simulink model "battery_PV_microgrid"  (R2014a)
settings: Solver=ode23tb  StartTime=0.0  StopTime=86000  MaxStep=0.2  RelTol=1e-5
InitFcn:
  | % Load Stateflow/Controller Parameters
  | controlParams();
  | 
  | % Load Initial Conditions for Model
  | initialConditions();
  | 
  | % Load Battery/PV Parameters
  | parameters();
StopFcn:
  | % Plot results
  | %plotSimResults();
values from neighbouring files (symbols this model uses):
  ambientTemp = 20    [initialConditions.m]    (also in initializeBattery.m)
  currentSat = 0.5    [controlParams.m]    (also in initializeBattery.m)
  desiredBusVoltage = 30    [controlParams.m]    (also in initializeBattery.m = 24.45)
  finalVoltage = 30    [controlParams.m]    (also in initializeBattery.m = 26)
  maxChargeRate = 5    [controlParams.m]    (also in initializeBattery.m)
  maxDischargeRate = -5    [controlParams.m]    (also in initializeBattery.m)
  Ncell = 100    [parameters.m]
  T_init = ambientTemp + 273.15    (= 293.15)    [initialConditions.m]    (also in initializeBattery.m)
  tau = 1e-4    (= 0.0001)    [parameters.m]
undefined symbols (not defined in the file or in its folder): hysteresisSOC, Ion, Lithium, maxSOC, minSOC, optTime, powerHysteresis
undefined symbols (not defined in the file): C1_LUT, C2_LUT, Capacity_LUT, cell_Cp_heat, cell_mass, Em_LUT, PVCellIsc, PVCellRs, PVCellVoc, Qe_init, R0_LUT, R1_LUT, R2_LUT, SOC_LUT, Temperature_LUT
libraries: powerlib x49, fl_lib x18, nesl_utility x6, LiBatteryElements_lib x6, simulink x3, simulink_extras x3, electricdrivelib x1
(part 1 of 2)
settings Model: Creator=jlesage  LastModifiedBy=jlesage
settings DataIOCC: LimitDataPoints=off
settings DebuggingCC: MergeDetectMultiDrivingBlocksExec=error
settings SimscapeCC: ExplicitSolverDiagnosticOptions=none

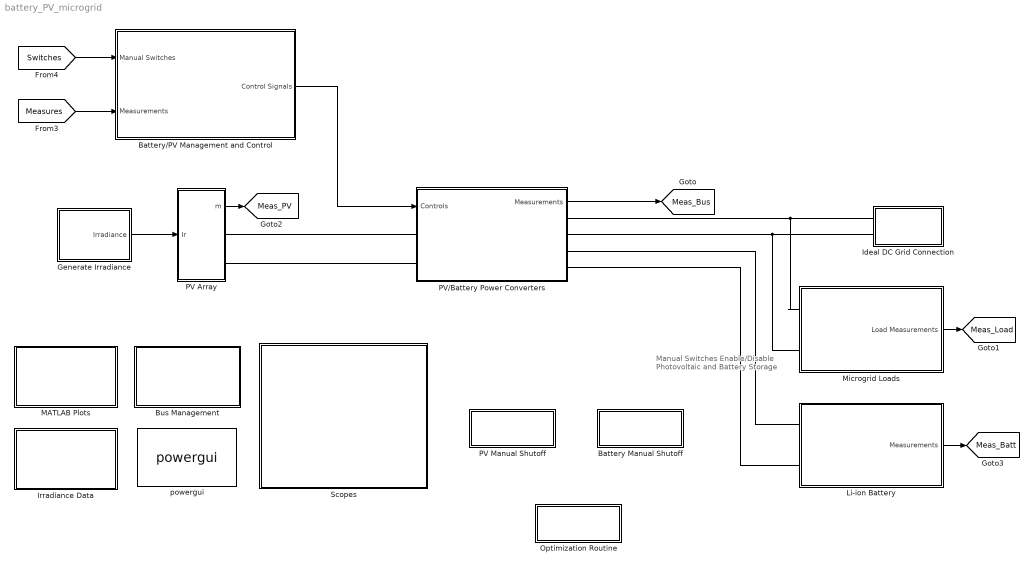
== system battery_PV_microgrid ==
  note: Manual Switches
      | Enable/Disable Photovoltaic
      | and Battery Storage
  Battery Manual Shutoff : Subsystem
      settings: OpenFcn=|
      | blkName = gcb;
      | switchBlkName = [gcb '/ControlValue'];
      | 
      | switchValue = get_param(switchBlkName,'Value');
      | switchValue = str2num(switchValue);
      | 
      | if switchValue > 0,
      | 
      | set_param(switchBlkName,'Value','-1');
      | set_param(blkName,'BackgroundColor','red');
      | set_param(blkName,'MaskDisplay','disp(''Battery On/Off\nOFF'')');
      | 
      | else
      | 
      | set_param(switchBlkName,'Value','1');
      | set_param(blkName,'BackgroundColor','green');
      | set_param(blkName,'MaskDisplay','disp(''Battery On/Off\nON'')');
      | 
      | 
      | end
      mask Display: disp('Battery On/Off\nON')
  Battery/PV Management and Control : Subsystem
  Bus Management : Subsystem
      mask Display: disp('Bus\nManagement');
  Generate Irradiance : Subsystem
  Ideal DC Grid Connection : Subsystem
  Irradiance Data : Subsystem
      settings: OpenFcn=|
      | blkName = gcb;
      | switchBlkName = [gcb '/ControlValue'];
      | 
      | switchValue = get_param(switchBlkName,'Value');
      | switchValue = str2num(switchValue);
      | 
      | if switchValue > 0,
      | 
      | set_param(switchBlkName,'Value','-1');
      | set_param(blkName,'MaskDisplay','disp(''Irradiance Data:\n Cloudy Day'')');
      | 
      | else
      | 
      | set_param(switchBlkName,'Value','1');
      | set_param(blkName,'MaskDisplay','disp(''Irradiance Data:\n Clear Day'')');
      | 
      | 
      | end
      mask Display: disp('Irradiance Data:\n Cloudy Day')
  Li-ion Battery : Subsystem  Variant=on  OverrideUsingVariant=Variant
  MATLAB Plots : Subsystem
      settings: OpenFcn=|
      | try
      | plotSimResults();
      | catch
      | disp('Run simulation before plotting results...');
      | end
      mask Display: disp('Plot Simulation\nResults');
  Microgrid Loads : Subsystem  Variant=on  OverrideUsingVariant=Variant
  Optimization Routine : Subsystem
      settings: OpenFcn=|
      | blkName = gcb;
      | switchBlkName = [gcb '/ControlValue'];
      | 
      | switchValue = get_param(switchBlkName,'Value');
      | switchValue = str2num(switchValue);
      | 
      | if switchValue > 0,
      | 
      | set_param(switchBlkName,'Value','-1');
      | set_param(blkName,'BackgroundColor','red');
      | set_param(blkName,'MaskDisplay','disp(''Optimization:\nOFF'')');
      | 
      | else
      | 
      | set_param(switchBlkName,'Value','1');
      | set_param(blkName,'BackgroundColor','green');
      | set_param(blkName,'MaskDisplay','disp(''Optimization:\nON'')');
      | 
      | 
      | end
      mask Display: disp('Optimization:\nOFF')
  PV Array : Subsystem
      mask Display: image(imread('panel.jpg'))
  PV Manual Shutoff : Subsystem
      settings: OpenFcn=|
      | blkName = gcb;
      | switchBlkName = [gcb '/ControlValue'];
      | 
      | switchValue = get_param(switchBlkName,'Value');
      | switchValue = str2num(switchValue);
      | 
      | if switchValue > 0,
      | 
      | set_param(switchBlkName,'Value','-1');
      | set_param(blkName,'BackgroundColor','red');
      | set_param(blkName,'MaskDisplay','disp(''PV On/Off\nOFF'')');
      | 
      | else
      | 
      | set_param(switchBlkName,'Value','1');
      | set_param(blkName,'BackgroundColor','green');
      | set_param(blkName,'MaskDisplay','disp(''PV On/Off\nON'')');
      | 
      | 
      | end
      mask Display: disp('PV On/Off\nON')
  PV/Battery Power Converters : Subsystem
  Scopes : Subsystem
      mask Display: disp('System\nMeasurements');
  powergui : powerlib/powergui  Priority=1  SimulationMode=Continuous  SolverType=Tustin  SampleTime=50e-6  frequency=60  SPID=on  DisableSnubberDevices=off  DisableRonSwitches=off  DisableVfSwitches=off  SwTol=0  Interpol=off  DisplayEquations=off  Ts=0  methode=off  frequencyindice=0  Pbase=100e6  ErrMax=1e-4  Iterations=50  UnitsV=kV  UnitsW=MW  FunctionMessages=off  echomessages=off  HookPort=off  EnableUseOfTLC=off  x0status=blocks  RestoreLinks=warning  ResistiveCurrentMeasurement=off  Frange=[0:2:500]  Ylog=off  Xlog=on  ShowGrid=off  save=off  variable=ZData  structure=0  ZoomFFT=off  StartTime=0.0  cycles=1  DisplayStyle=1  fundamental=60  FreqAxis=off  MaxFrequency=1000  frequencyindicesteady=1  RmsSteady=1  display=off
  tag scope: Meas_Batt=global, Meas_Bus=global, Meas_Load=global, Meas_PV=global
  wires:
  Microgrid Loads/1(Load Measurements) -> [Meas_Load]
  PV Array/1(m) -> [Meas_PV]
  Generate Irradiance/1(Irradiance) -> PV Array/1(Ir)
  Li-ion Battery/1(Measurements) -> [Meas_Batt]
  [Measures] -> Battery/PV Management and Control/2(Measurements)
  Battery/PV Management and Control/1(Control Signals) -> PV/Battery Power Converters/1(Controls)
  PV/Battery Power Converters/1(Measurements) -> [Meas_Bus]
  [Switches] -> Battery/PV Management and Control/1(Manual Switches)
  connections:
  Microgrid Loads/LConn2 -- PV/Battery Power Converters/RConn2 -- Ideal DC Grid Connection/LConn2
  Microgrid Loads/LConn1 -- PV/Battery Power Converters/RConn1 -- Ideal DC Grid Connection/LConn1
  PV Array/RConn1 -- PV/Battery Power Converters/LConn1
  PV Array/RConn2 -- PV/Battery Power Converters/LConn2
  PV/Battery Power Converters/RConn3 -- Li-ion Battery/LConn1
  Li-ion Battery/LConn2 -- PV/Battery Power Converters/RConn4

== system battery_PV_microgrid/Battery Manual Shutoff ==
  ControlValue : Constant
  Off : Constant  Value=0
  On : Constant
  Switch : Switch
  tag scope: BatterySwitch=global
  wires:
  Off/1 -> Switch/3
  ControlValue/1 -> Switch/2
  On/1 -> Switch/1
  Switch/1 -> [BatterySwitch]

== system battery_PV_microgrid/Battery//PV Management and Control ==
  Manual Switches : Inport
  Measurements : Inport  Port=2
  Battery Charge/Discharge Controllers : Subsystem
  Battery Mode Selection : Stateflow chart  TreatAsAtomicUnit=on
  Bus Creator : BusCreator  OutDataTypeStr=Bus: Controls
  Bus Selector : BusSelector  OutputSignals=pv
  Bus Selector1 : BusSelector  Commented=on  OutputSignals=opt
  MPPT Algorithm : Subsystem
  Optimization Routine : Subsystem  Commented=on  TreatAsAtomicUnit=on
  Signal Conversion : SignalConversion
  Control Signals : Outport
  tag scope: gridOnOff=global
  wires:
  Manual Switches/1 -> Bus Selector1/1, Bus Selector/1, Battery Mode Selection/1(switches)
  Battery Charge/Discharge Controllers/1(Duty) -> Bus Creator/3  "dutyBatt"
  Battery Mode Selection/1(controlOnOff) -> Battery Charge/Discharge Controllers/Enable, Bus Creator/2  "enableBatt"
  Bus Creator/1 -> Control Signals/1
  Battery Mode Selection/3(controlSelect) -> Battery Charge/Discharge Controllers/2(Controller Mode)
  Battery Mode Selection/2(batteryMode) -> Battery Charge/Discharge Controllers/1(Bus Switch)
  MPPT Algorithm/1(PV Duty) -> Bus Creator/4  "dutyPV"
  Bus Selector/1 -> Signal Conversion/1  "<pv>"
  Signal Conversion/1 -> Bus Creator/1  "enablePV"
  Battery Mode Selection/4(gridOnOff) -> [gridOnOff]
  Measurements/1 -> Optimization Routine/1(In1), MPPT Algorithm/1(Measurements), Battery Charge/Discharge Controllers/3(Measurements), Battery Mode Selection/2(measures)
  Bus Selector1/1 -> Optimization Routine/Enable  "<opt>"

== system battery_PV_microgrid/Bus Management ==
  note: Measurement Bus
  note: Manual Switch Bus
  note: ff
  note: ff
  note: Construct Measurement and Switch Buses
  Bus Creator : BusCreator  Inputs=5  OutDataTypeStr=Bus: Measurements
  Bus Creator1 : BusCreator  Inputs=3  OutDataTypeStr=Bus: Switches
  tag scope: Measures=global, Switches=global
  wires:
  [Meas_Load] -> Bus Creator/3  "load"
  [Meas_Bus] -> Bus Creator/2  "bus"
  Bus Creator/1 -> [Measures]
  [Meas_Batt] -> Bus Creator/5  "batt"
  [Meas_PV] -> Bus Creator/4  "pv"
  [BatterySwitch] -> Bus Creator1/2  "battery"
  [PVSwitch] -> Bus Creator1/1  "pv"
  Bus Creator1/1 -> [Switches]  "switches"
  [Meas_Grid] -> Bus Creator/1  "grid"
  [OptSwitch] -> Bus Creator1/3  "opt"

== system battery_PV_microgrid/Generate Irradiance ==
  Constant : Constant  Value=10
  From Workspace : FromWorkspace  VariableName=clearIrrad  SampleTime=0
  From Workspace1 : FromWorkspace  VariableName=cloudyIrrad  SampleTime=0
  Irradiance Data : Scope
      settings: TimeRange=4000  YMin=0  YMax=450  SaveName=irradiance
  Logic : Switch  Criteria=u2 > Threshold  Threshold=10
  Low-pass : TransferFcn  Numerator=5  Denominator=[1 5]
  Switch : Switch  Criteria=u2 > Threshold
  Irradiance : Outport
  wires:
  Low-pass/1 -> Logic/1, Logic/2, Irradiance Data/1
  Logic/1 -> Irradiance/1
  Constant/1 -> Logic/3
  From Workspace/1 -> Switch/1
  Switch/1 -> Low-pass/1
  [selectIrradiance] -> Switch/2
  From Workspace1/1 -> Switch/3

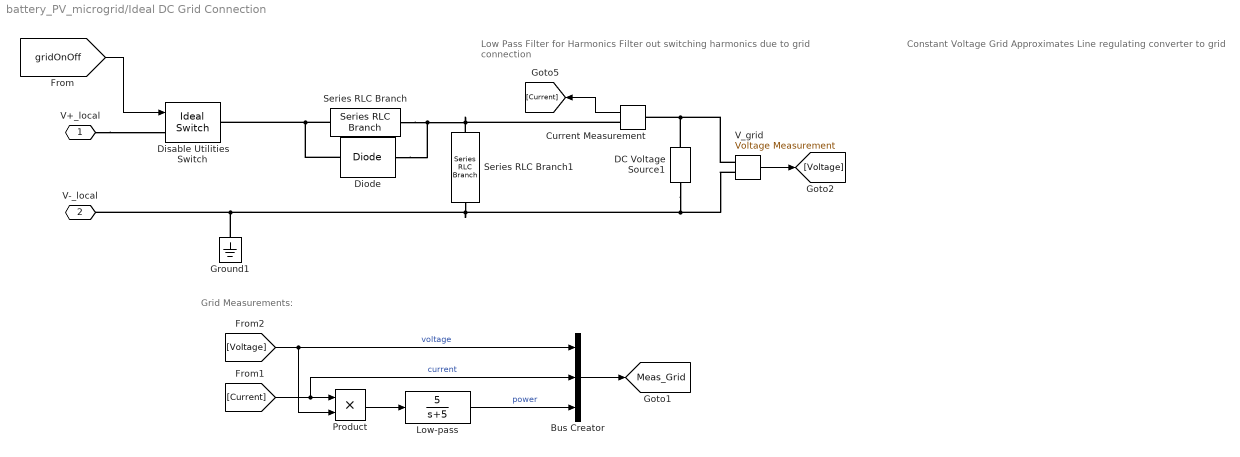
== system battery_PV_microgrid/Ideal DC Grid Connection ==
  note: Constant Voltage Grid
      | Approximates Line regulating converter to grid
  note: Grid Measurements:
  note: Low Pass Filter for Harmonics
      | Filter out switching harmonics due to grid connection
  Bus Creator : BusCreator  Inputs=3  OutDataTypeStr=Bus: Grid
  Current Measurement : powerlib/Measurements/Current Measurement  PhasorSimulation=off  OutputType=Complex  PSBequivalent=0
  DC Voltage Source1 : powerlib/Electrical Sources/DC Voltage Source  Amplitude=desiredBusVoltage  Measurements=None
  Diode : powerlib/Power Electronics/Diode  Ron=0.001  Lon=0  Vf=0.8  IC=0  UseSnubber=off  Rs=500  Cs=250e-9  Measurements=off
  Disable Utilities Switch : powerlib/Power Electronics/Ideal Switch  Ron=1e-6  Lon=0  IC=0  Rs=inf  Cs=inf  Measurements=off
  Ground1 : powerlib/Elements/Ground  LConnTagsString=a
  Low-pass : TransferFcn  Numerator=[5]  Denominator=[1 5]
  Product : Product
  Series RLC Branch : powerlib/Elements/Series RLC Branch  LConnTagsString=__new0  RConnTagsString=__new0  BranchType=L  Resistance=1  Inductance=5e-2  SetiL0=on  InitialCurrent=-3  Capacitance=1e-6  Setx0=off  InitialVoltage=0  Measurements=None
  Series RLC Branch1 : powerlib/Elements/Series RLC Branch  LConnTagsString=__new0  RConnTagsString=__new0  BranchType=RC  Resistance=0.01  Inductance=1e-3  SetiL0=off  InitialCurrent=0  Capacitance=1e-3  Setx0=off  InitialVoltage=0  Measurements=None
  V_grid : powerlib/Measurements/Voltage Measurement  PhasorSimulation=off  OutputType=Complex  PSBequivalent=0
  V+_local : PMIOPort  Port=1  Side=Left
  V-_local : PMIOPort  Port=2  Side=Left
  tag scope: Meas_Grid=global
  wires:
  [Voltage] -> Bus Creator/1, Product/2  "voltage"
  Product/1 -> Low-pass/1
  Bus Creator/1 -> [Meas_Grid]
  Low-pass/1 -> Bus Creator/3  "power"
  [gridOnOff] -> Disable Utilities Switch/1
  Current Measurement/1 -> [Current]
  [Current] -> Bus Creator/2, Product/1  "current"
  V_grid/1 -> [Voltage]
  connections:
  V+_local/RConn1 -- Disable Utilities Switch/LConn1
  V_grid/LConn2 -- DC Voltage Source1/LConn1 -- Series RLC Branch1/RConn1 -- Ground1/LConn1 -- V-_local/RConn1
  V_grid/LConn1 -- DC Voltage Source1/RConn1 -- Current Measurement/LConn1
  Series RLC Branch/RConn1 -- Diode/RConn1 -- Current Measurement/RConn1 -- Series RLC Branch1/LConn1
  Series RLC Branch/LConn1 -- Diode/LConn1 -- Disable Utilities Switch/RConn1

== system battery_PV_microgrid/Irradiance Data ==
  Clear Day : Constant
  Cloudy Day : Constant  Value=0
  ControlValue : Constant  Value=-1
  Switch : Switch
  tag scope: selectIrradiance=global
  wires:
  Clear Day/1 -> Switch/1
  ControlValue/1 -> Switch/2
  Cloudy Day/1 -> Switch/3
  Switch/1 -> [selectIrradiance]

== system battery_PV_microgrid/Li-ion Battery ==
  note: Li-ion Battery Models
      | 1) SimPowerSystems Specialized Technology
      | 2) Simscape Li-ion equivalent circuit
  SimPowerSystems Model : Subsystem  VariantControl=(default)
  Simscape Li-ion Model : Subsystem  VariantControl=Variant
  V_battery+ : PMIOPort  Port=1  Side=Left
  V_battery- : PMIOPort  Port=2  Side=Left
  Measurements : Outport

== system battery_PV_microgrid/MATLAB Plots ==

== system battery_PV_microgrid/Microgrid Loads ==
  Ideal Constant Resistance Load : Subsystem  VariantControl=(default)
  Ideal Constant Power Load : Subsystem  VariantControl=Variant
  V_P+ : PMIOPort  Port=1  Side=Left
  V_P- : PMIOPort  Port=2  Side=Left
  Load Measurements : Outport

== system battery_PV_microgrid/Optimization Routine ==
  ControlValue : Constant  Value=-1
  Off : Constant  Value=0
  On : Constant
  Switch : Switch
  tag scope: OptSwitch=global
  wires:
  Switch/1 -> [OptSwitch]
  Off/1 -> Switch/3
  ControlValue/1 -> Switch/2
  On/1 -> Switch/1

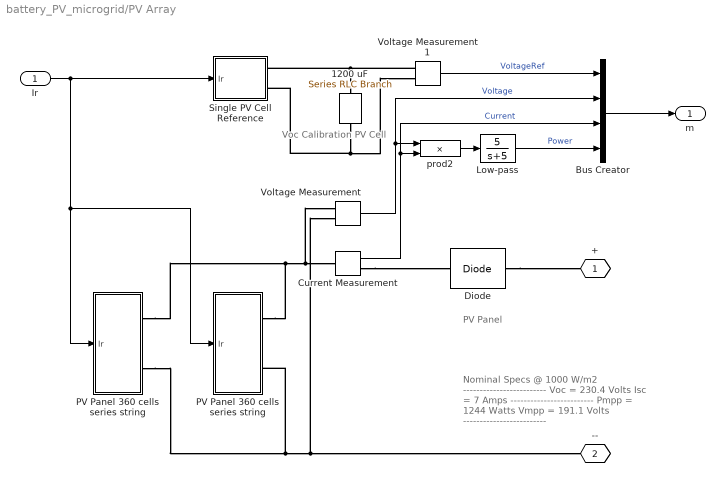
== system battery_PV_microgrid/PV Array ==
  note: Voc Calibration PV Cell
  note: Nominal Specs @ 1000 W/m2
      | -------------------------
      | Voc = 230.4 Volts
      | Isc = 7 Amps
      | -------------------------
      | Pmpp = 1244 Watts
      | Vmpp = 191.1 Volts
      | -------------------------
  note: PV Panel
  Ir : Inport
  1200 uF : powerlib/Elements/Series RLC Branch  LConnTagsString=__new0  RConnTagsString=__new0  BranchType=C  Resistance=0.05  Inductance=1e-3  SetiL0=off  InitialCurrent=0  Capacitance=1200e-6  Setx0=on  InitialVoltage=PVCellVoc  Measurements=None
  Bus Creator : BusCreator  OutDataTypeStr=Bus: PV
  Current Measurement : powerlib/Measurements/Current Measurement  PhasorSimulation=off  OutputType=Complex  PSBequivalent=0
  Diode : powerlib/Power Electronics/Diode  Ron=0.001  Lon=0  Vf=0.8  IC=0  UseSnubber=off  Rs=500  Cs=250e-9  Measurements=off
  Low-pass : TransferFcn  Numerator=[5]  Denominator=[1 5]
  PV Panel 360 cells series string : Subsystem  mask(Solar Cell){Isc=PVCellIsc, Voc=PVCellVoc*Ncell, Ir0=1000, N=1.5*Ncell, Rs=PVCellRs*Ncell, Rp=1000*Ncell, tau=tau}
      mask prompts: Isc "Short-circuit current, Isc (A):"; Voc "Open-circuit voltage, Voc (V):"; Ir0 "Irradiance used for measurements, Ir0 (W/m2):"; N "Quality factor, N:"; Rs "Series resistance, Rs (ohms):"; Rp "Parallel resistance, Rp (ohms):"; tau "Time constant (sec):"
      mask help:
      | Simulink implementation of an idividual solar cell. The cell is modelled as a parallel combination of a current source, an exponential diode and an internal resistance Rp, connected in series with a resistance Rs.
      | The cell output current is given by:
      |
      | Ipv = Iph - Is * (exp((V + I*Rs)/(N*Vt)) - 1) - (V + I*Rs)/Rp
      |
      | Where Iph is the solar generated current, Is is the diode saturation current, Vt is the thermal voltage, N is the diode quality factor (emission coefficient).
      |
      | A first order transfer function is used to break the algebraic loop. The time constant of this transfer function should be adjusted such that it will not significantly affect your model dynamics.
      mask init:
      | %% Cell thermal voltage calculation
      | T = 25 + 273;   % Device operating temperature (oC)
      | k = 1.3806e-23; % Boltzman constant (J/oK)
      | q = 1.602e-19;  % Elementary charge on an electron (oC)
      | Vt = k*T/q;     % Thermal voltage
      | 
      | %% Diode saturation current calculation
      | Is = Isc/(exp(Voc/(N*Vt))-1);
  "PV Panel 360 cells series string " : Subsystem  mask(Solar Cell){Isc=PVCellIsc, Voc=PVCellVoc*Ncell, Ir0=1000, N=1.5*Ncell, Rs=PVCellRs*Ncell, Rp=1000*Ncell, tau=tau}
      mask prompts: Isc "Short-circuit current, Isc (A):"; Voc "Open-circuit voltage, Voc (V):"; Ir0 "Irradiance used for measurements, Ir0 (W/m2):"; N "Quality factor, N:"; Rs "Series resistance, Rs (ohms):"; Rp "Parallel resistance, Rp (ohms):"; tau "Time constant (sec):"
      mask help:
      | Simulink implementation of an idividual solar cell. The cell is modelled as a parallel combination of a current source, an exponential diode and an internal resistance Rp, connected in series with a resistance Rs.
      | The cell output current is given by:
      |
      | Ipv = Iph - Is * (exp((V + I*Rs)/(N*Vt)) - 1) - (V + I*Rs)/Rp
      |
      | Where Iph is the solar generated current, Is is the diode saturation current, Vt is the thermal voltage, N is the diode quality factor (emission coefficient).
      |
      | A first order transfer function is used to break the algebraic loop. The time constant of this transfer function should be adjusted such that it will not significantly affect your model dynamics.
      mask init: same as battery_PV_microgrid/PV Array/PV Panel 360 cells series string
  Single PV Cell Reference : Subsystem  mask(Solar Cell){Isc=PVCellIsc, Voc=PVCellVoc, Ir0=1000, N=1.5, Rs=PVCellRs, Rp=1000, tau=tau}
      mask prompts: Isc "Short-circuit current, Isc (A):"; Voc "Open-circuit voltage, Voc (V):"; Ir0 "Irradiance used for measurements, Ir0 (W/m2):"; N "Quality factor, N:"; Rs "Series resistance, Rs (ohms):"; Rp "Parallel resistance, Rp (ohms):"; tau "Time constant (sec):"
      mask help:
      | Simulink implementation of an idividual solar cell. The cell is modelled as a parallel combination of a current source, an exponential diode and an internal resistance Rp, connected in series with a resistance Rs.
      | The cell output current is given by:
      |
      | Ipv = Iph - Is * (exp((V + I*Rs)/(N*Vt)) - 1) - (V + I*Rs)/Rp
      |
      | Where Iph is the solar generated current, Is is the diode saturation current, Vt is the thermal voltage, N is the diode quality factor (emission coefficient).
      |
      | A first order transfer function is used to break the algebraic loop. The time constant of this transfer function should be adjusted such that it will not significantly affect your model dynamics.
      mask init: same as battery_PV_microgrid/PV Array/PV Panel 360 cells series string
  Voltage Measurement : powerlib/Measurements/Voltage Measurement  PhasorSimulation=off  OutputType=Complex  PSBequivalent=0
  Voltage Measurement1 : powerlib/Measurements/Voltage Measurement  PhasorSimulation=off  OutputType=Complex  PSBequivalent=0
  prod2 : Product  Inputs=**
  + : PMIOPort  Tag=PMCPort  Port=1  Side=Right
  -- : PMIOPort  Tag=PMCPort  Port=2  Side=Right
  m : Outport
  wires:
  prod2/1 -> Low-pass/1
  Current Measurement/1 -> prod2/2, Bus Creator/3  "Current"
  Voltage Measurement1/1 -> Bus Creator/1  "VoltageRef"
  Ir/1 -> PV Panel 360 cells series string/1(Ir), "PV Panel 360 cells series string "/1(Ir), Single PV Cell Reference/1(Ir)
  Bus Creator/1 -> m/1
  Voltage Measurement/1 -> prod2/1, Bus Creator/2  "Voltage"
  Low-pass/1 -> Bus Creator/4  "Power"
  connections:
  Single PV Cell Reference/RConn1 -- 1200 uF/LConn1 -- Voltage Measurement1/LConn1
  Single PV Cell Reference/RConn2 -- Voltage Measurement1/LConn2 -- 1200 uF/RConn1
  "PV Panel 360 cells series string "/RConn2 -- --/RConn1 -- Voltage Measurement/LConn2 -- PV Panel 360 cells series string/RConn2
  "PV Panel 360 cells series string "/RConn1 -- Current Measurement/LConn1 -- Voltage Measurement/LConn1 -- PV Panel 360 cells series string/RConn1
  Current Measurement/RConn1 -- Diode/LConn1
  Diode/RConn1 -- +/RConn1

== system battery_PV_microgrid/PV Manual Shutoff ==
  ControlValue : Constant
  Off : Constant  Value=0
  On : Constant
  Switch : Switch
  tag scope: PVSwitch=global
  wires:
  On/1 -> Switch/1
  ControlValue/1 -> Switch/2
  Off/1 -> Switch/3
  Switch/1 -> [PVSwitch]

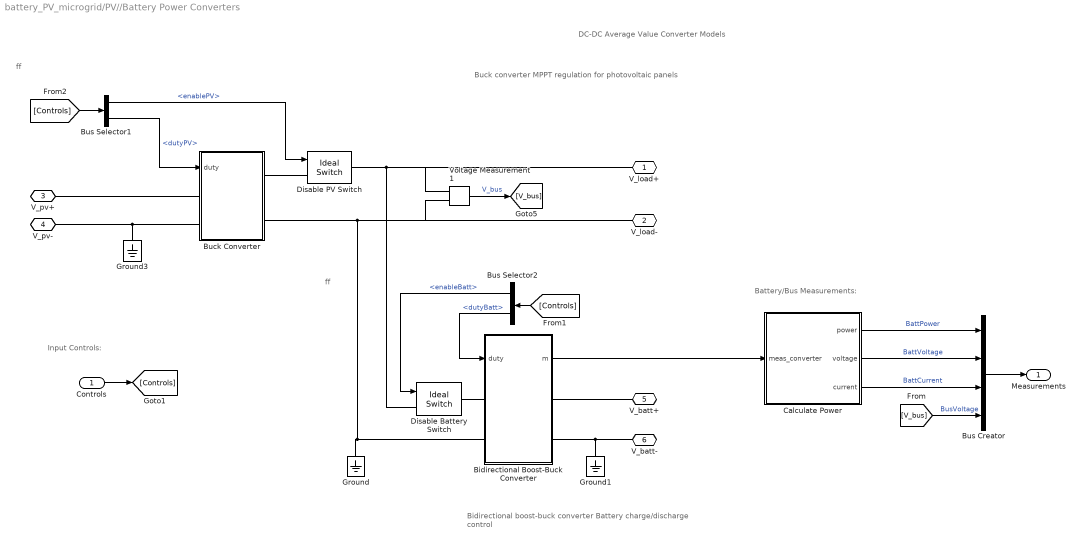
== system battery_PV_microgrid/PV//Battery Power Converters ==
  note: Bidirectional boost-buck converter
      | Battery charge/discharge control
  note: Buck converter
      | MPPT regulation for photovoltaic panels
  note: ff
  note: DC-DC Average Value Converter Models
  note: ff
  note: Input Controls:
  note: Battery/Bus Measurements:
  Controls : Inport
  Bidirectional Boost-Buck Converter : Subsystem  VariantControl=DCDCBuckAVG
  Buck Converter : Subsystem  VariantControl=DCDCBuckAVG
  Bus Creator : BusCreator  OutDataTypeStr=Bus: Bus
  Bus Selector1 : BusSelector  OutputSignals=enablePV,dutyPV
  Bus Selector2 : BusSelector  OutputSignals=enableBatt,dutyBatt
  Calculate Power : Subsystem
  Disable Battery Switch : powerlib/Power Electronics/Ideal Switch  Ron=0.001  Lon=0  IC=0  Rs=1e5  Cs=inf  Measurements=off
  Disable PV Switch : powerlib/Power Electronics/Ideal Switch  Ron=1e-6  Lon=0  IC=0  Rs=inf  Cs=inf  Measurements=off
  Ground : powerlib/Elements/Ground  LConnTagsString=a
  Ground1 : powerlib/Elements/Ground  LConnTagsString=a
  Ground3 : powerlib/Elements/Ground  LConnTagsString=a
  Voltage Measurement1 : powerlib/Measurements/Voltage Measurement  PhasorSimulation=off  OutputType=Complex  PSBequivalent=0
  V_load+ : PMIOPort  Port=1  Side=Right
  V_load- : PMIOPort  Port=2  Side=Right
  V_pv+ : PMIOPort  Port=3  Side=Left
  V_pv- : PMIOPort  Port=4  Side=Left
  V_batt+ : PMIOPort  Port=5  Side=Right
  V_batt- : PMIOPort  Port=6  Side=Right
  Measurements : Outport
  wires:
  Voltage Measurement1/1 -> [V_bus]  "V_bus"
  [V_bus] -> Bus Creator/4  "BusVoltage"
  Bus Selector2/2 -> Bidirectional Boost-Buck Converter/1(duty)  "<dutyBatt>"
  Bus Selector2/1 -> Disable Battery Switch/1  "<enableBatt>"
  Bus Selector1/2 -> Buck Converter/1(duty)  "<dutyPV>"
  Bus Creator/1 -> Measurements/1
  Calculate Power/1(power) -> Bus Creator/1  "BattPower"
  Calculate Power/3(current) -> Bus Creator/3  "BattCurrent"
  Calculate Power/2(voltage) -> Bus Creator/2  "BattVoltage"
  Bidirectional Boost-Buck Converter/1(m) -> Calculate Power/1(meas_converter)
  Controls/1 -> [Controls]
  [Controls] -> Bus Selector2/1
  [Controls] -> Bus Selector1/1
  Bus Selector1/1 -> Disable PV Switch/1  "<enablePV>"
  connections:
  Bidirectional Boost-Buck Converter/RConn2 -- V_batt-/RConn1 -- Ground1/LConn1
  Disable Battery Switch/RConn1 -- Bidirectional Boost-Buck Converter/LConn1
  V_pv+/RConn1 -- Buck Converter/LConn1
  Buck Converter/LConn2 -- V_pv-/RConn1 -- Ground3/LConn1
  Disable PV Switch/LConn1 -- Buck Converter/RConn1
  Voltage Measurement1/LConn1 -- V_load+/RConn1 -- Disable Battery Switch/LConn1 -- Disable PV Switch/RConn1
  Bidirectional Boost-Buck Converter/RConn1 -- V_batt+/RConn1
  Bidirectional Boost-Buck Converter/LConn2 -- Buck Converter/RConn2 -- Voltage Measurement1/LConn2 -- V_load-/RConn1 -- Ground/LConn1

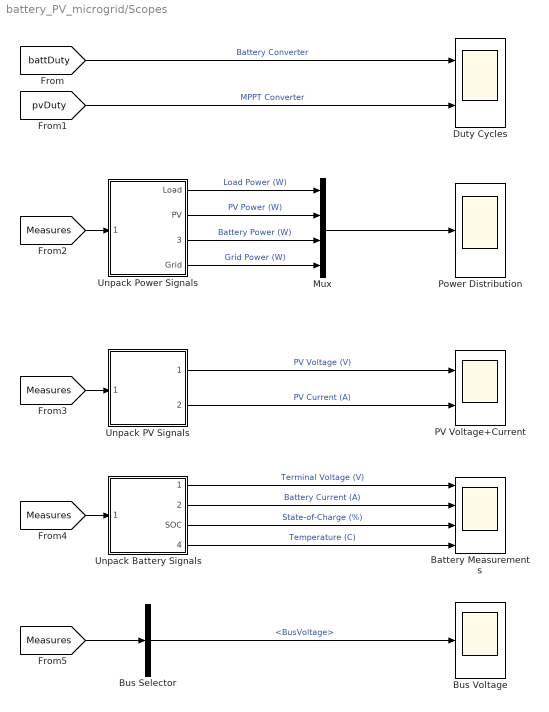
== system battery_PV_microgrid/Scopes ==
  Battery Measurements : Scope  NumInputPorts=4
      settings: TimeRange=50000  YMin=18~-40~0~20  YMax=28~40~100~24  SaveName=BatteryData
  Bus Selector : BusSelector  OutputSignals=bus.BusVoltage
  Bus Voltage : Scope
      settings: ShowLegends=on  TimeRange=3500  YMin=28.5  YMax=31.5  SaveName=duty3  DataFormat=Structure
  Duty Cycles : Scope  NumInputPorts=2
      settings: TimeRange=4000  YMin=-0.05~-0.3  YMax=1~0.225  SaveName=duty
  Mux : Mux
  PV Voltage+Current : Scope  NumInputPorts=2
      settings: TimeRange=3500  YMin=20~-20  YMax=60~15  SaveName=duty5  DataFormat=Structure
  Power Distribution : Scope
      settings: ShowLegends=on  TimeRange=90000  YMin=-800  YMax=1000  SaveName=PowerDist
  Unpack Battery Signals : Subsystem
  Unpack PV Signals : Subsystem
  Unpack Power Signals : Subsystem
  wires:
  [battDuty] -> Duty Cycles/1  "Battery Converter"
  [pvDuty] -> Duty Cycles/2  "MPPT Converter"
  Mux/1 -> Power Distribution/1
  Unpack Power Signals/1(Load) -> Mux/1  "Load Power (W)"
  Unpack Power Signals/2(PV) -> Mux/2  "PV Power (W)"
  Unpack Power Signals/3(Battery) -> Mux/3  "Battery Power (W)"
  [Measures] -> Unpack Power Signals/1(Measure)
  [Measures] -> Unpack PV Signals/1(Measure)
  Unpack PV Signals/1(Voltage) -> PV Voltage+Current/1  "PV Voltage (V)"
  Unpack PV Signals/2(Current) -> PV Voltage+Current/2  "PV Current (A)"
  [Measures] -> Unpack Battery Signals/1(Measure)
  Unpack Battery Signals/1(Voltage) -> Battery Measurements/1  "Terminal Voltage (V)"
  Unpack Battery Signals/2(Current) -> Battery Measurements/2  "Battery Current (A)"
  Unpack Battery Signals/4(Temperature) -> Battery Measurements/4  "Temperature (C)"
  Unpack Battery Signals/3(SOC) -> Battery Measurements/3  "State-of-Charge (%)"
  [Measures] -> Bus Selector/1
  Bus Selector/1 -> Bus Voltage/1  "<BusVoltage>"
  Unpack Power Signals/4(Grid) -> Mux/4  "Grid Power (W)"

== system battery_PV_microgrid/Battery//PV Management and Control/Battery Charge//Discharge Controllers ==
  Bus Switch : Inport
  Controller Mode : Inport  Port=2
  Measurements : Inport  Port=3
  Enable : EnablePort  StatesWhenEnabling=reset
  Battery Charge Controller : Subsystem
  Battery Discharge Controller : Subsystem
  Merge : Merge
  Switch Case : SwitchCase
  Duty : Outport  InitialOutput=0
  wires:
  Battery Discharge Controller/1(Duty) -> Merge/2
  Battery Charge Controller/1(Duty) -> Merge/1
  Merge/1 -> Duty/1
  Bus Switch/1 -> Switch Case/1
  Controller Mode/1 -> Battery Discharge Controller/1(Controller Mode), Battery Charge Controller/1(Controller Mode)
  Measurements/1 -> Battery Charge Controller/2(Measurements), Battery Discharge Controller/2(Measurements)
  Switch Case/1 -> [Charge]
  [Charge] -> Battery Charge Controller/Action
  Switch Case/2 -> [Discharge]
  [Discharge] -> Battery Discharge Controller/Action

== system battery_PV_microgrid/Battery//PV Management and Control/MPPT Algorithm ==
  note: Fractional Open Circuit Voltage Algorithm
  Measurements : Inport
  # of cells in series : Gain  Gain=Ncell
  Bus Selector3 : BusSelector  OutputSignals=pv.VoltageRef,pv.Voltage
  Divide : Product  Inputs=*/
  MPP fraction : Gain  Gain=0.82
  PI Controller : simulink/Continuous/PID Controller  Controller=PI  TimeDomain=Continuous-time  SampleTime=-1  IntegratorMethod=Forward Euler  FilterMethod=Forward Euler  Form=Parallel  P=1  I=2.5  D=2  N=100  InitialConditionSource=internal  InitialConditionForIntegrator=0  InitialConditionForFilter=0  ExternalReset=none  LimitOutput=on  UpperSaturationLimit=40  LowerSaturationLimit=0  LinearizeAsGain=off  AntiWindupMode=back-calculation  Kb=1  TrackingMode=off  Kt=1  PParamMin=[]  PParamMax=[]  IParamMin=[]  IParamMax=[]  DParamMin=[]  DParamMax=[]  NParamMin=[]  NParamMax=[]  KbParamMin=[]  KbParamMax=[]  KtParamMin=[]  KtParamMax=[]  POutMin=[]  POutMax=[]  IOutMin=[]  IOutMax=[]  DOutMin=[]  DOutMax=[]  NOutMin=[]  NOutMax=[]  KbOutMin=[]  KbOutMax=[]  KtOutMin=[]  KtOutMax=[]  IntegratorOutMin=[]  IntegratorOutMax=[]  FilterOutMin=[]  FilterOutMax=[]  SumOutMin=[]  SumOutMax=[]  SumI1OutMin=[]  SumI1OutMax=[]  SumI2OutMin=[]  SumI2OutMax=[]  SumI3OutMin=[]  SumI3OutMax=[]  SumDOutMin=[]  SumDOutMax=[]  SaturationOutMin=[]  SaturationOutMax=[]  IntegratorContinuousStateAttributes=''  IntegratorStateMustResolveToSignalObject=off  IntegratorRTWStateStorageClass=Auto  FilterContinuousStateAttributes=''  FilterStateMustResolveToSignalObject=off  FilterRTWStateStorageClass=Auto
  Saturation [0...1] : Saturate  UpperLimit=1  LowerLimit=0
  Scope : Scope  NumInputPorts=3
      settings: YMin=0~35~12.5  YMax=40~60~60  SaveName=ScopeData2
  Sum1 : Sum  Inputs=|-+
  PV Duty : Outport
  wires:
  Sum1/1 -> PI Controller/1  "Vdc_err"
  MPP fraction/1 -> Scope/3, Sum1/1  "Vdc*"
  # of cells in series/1 -> MPP fraction/1  "stringVoc"
  PI Controller/1 -> Scope/1, Divide/1
  Bus Selector3/2 -> Scope/2, Divide/2, Sum1/2  "<Voltage>"
  Bus Selector3/1 -> # of cells in series/1  "<VoltageRef>"
  Saturation [0...1]/1 -> PV Duty/1  "PV Duty"
  Divide/1 -> Saturation [0...1]/1
  Measurements/1 -> Bus Selector3/1

== system battery_PV_microgrid/Battery//PV Management and Control/Optimization Routine ==
  In1 : Inport
  Enable : EnablePort
  MATLAB Function : MATLAB Function  TreatAsAtomicUnit=on  SystemSampleTime=optTime
  Out1 : Outport
  wires:
  In1/1 -> MATLAB Function/1(u)
  MATLAB Function/1(y) -> Out1/1

== system battery_PV_microgrid/Li-ion Battery/SimPowerSystems Model ==
  Ambient Temperature : Constant  Value=ambientTemp
  Battery : electricdrivelib/Extra Sources/Battery  BatType=Lithium-Ion  ShowDetailedParameters=off  NomV=24  NomQ=6.5  SOC=40  PresetModel=on  MaxQ=6.5  FullV=27.9357  Dis_rate=2.8261  R=0.036923  Normal_OP=5.8783  expZone="[25.9293     0.319348]"  Dis_Char=off  current=[6.5 13 32.5]  Units=Time  Batt_Tr=30
  Bus Creator : BusCreator  OutDataTypeStr=Bus: Battery
  Bus Selector : BusSelector  OutputSignals=SOC (%),Current (A),Voltage (V)
  Signal Conversion : SignalConversion
  Signal Conversion1 : SignalConversion
  Signal Conversion2 : SignalConversion
  V_battery+ : PMIOPort  Port=1  Side=Left
  V_battery- : PMIOPort  Port=2  Side=Left
  Measurements : Outport
  wires:
  Ambient Temperature/1 -> Bus Creator/4  "Temperature"
  Battery/1 -> Bus Selector/1
  Bus Selector/1 -> Signal Conversion/1  "<SOC (%)>"
  Bus Selector/2 -> Signal Conversion1/1  "<Current (A)>"
  Bus Selector/3 -> Signal Conversion2/1  "<Voltage (V)>"
  Bus Creator/1 -> Measurements/1
  Signal Conversion/1 -> Bus Creator/1  "SOC"
  Signal Conversion1/1 -> Bus Creator/2  "Current"
  Signal Conversion2/1 -> Bus Creator/3  "Voltage"
  connections:
  V_battery+/RConn1 -- Battery/LConn1
  V_battery-/RConn1 -- Battery/LConn2

== system battery_PV_microgrid/Li-ion Battery/Simscape Li-ion Model ==
  note: Passive Low-pass Filter
      | Decrease transient current spikes on battery
  note: Simscape Battery Model
      | Simscape Interface converts from SimPowerSystems to Simscape
  note: ff
  note: Li-ion Battery Equivalent Circuit Model
  note: Battery Measurements:
  note: For the defining equations and their validation, see T. Huria, M. Ceraolo, J. Gazzarri, R. Jackey. "High Fidelity Electrical
      | Model with Thermal Dependence for Characterization and Simulation of High Power Lithium Battery Cells," IEEE International Electric Vehicle
      | Conference, March 2012. A simple thermal model is used to model battery temperature. It is assumed that cooling is primarily via convection,
      | and that heating is primarily from internal resistance. A battery pack can be modeled by connecting multiple copies of the battery cell block
      | in series.
  Ambient Temperature1 : Constant  Value=ambientTemp
  Bus Creator : BusCreator  OutDataTypeStr=Bus: Battery
  Ground : powerlib/Elements/Ground  LConnTagsString=a
  Li-Ion Battery : Subsystem
  Series RLC Branch1 : powerlib/Elements/Series RLC Branch  LConnTagsString=__new0  RConnTagsString=__new0  BranchType=RC  Resistance=0.1  Inductance=1e-3  SetiL0=off  InitialCurrent=0  Capacitance=1e-6  Setx0=off  InitialVoltage=0  Measurements=None
  Series RLC Branch4 : powerlib/Elements/Series RLC Branch  LConnTagsString=__new0  RConnTagsString=__new0  BranchType=RL  Resistance=0.1  Inductance=100e-6  SetiL0=off  InitialCurrent=0  Capacitance=1e-6  Setx0=off  InitialVoltage=0  Measurements=None
  To Percent : Gain  Gain=100
  Voltage-Current Simscape Interface : powerlib/Interface Elements/Voltage-Current Simscape Interface  DFT=off  Fmode=Second-order input filtering  T=1e-6  Ts=50e-6  i0=0  v0=0  Sd=SimPowerSystems side  Measurements=off
  V_battery+ : PMIOPort  Port=1  Side=Left
  V_battery- : PMIOPort  Port=2  Side=Left
  Measurements : Outport
  wires:
  [SOC] -> To Percent/1
  Ambient Temperature1/1 -> Li-Ion Battery/1(Ambient Temperature)
  To Percent/1 -> Bus Creator/1  "SOC"
  [I_load] -> Bus Creator/2  "Current"
  [V_load] -> Bus Creator/3  "Voltage"
  [T] -> Bus Creator/4  "Temperature"
  Bus Creator/1 -> Measurements/1
  connections:
  Voltage-Current Simscape Interface/RConn1 -- Li-Ion Battery/LConn1
  Voltage-Current Simscape Interface/RConn2 -- Li-Ion Battery/LConn2
  V_battery-/RConn1 -- Ground/LConn1 -- Series RLC Branch1/RConn1 -- Voltage-Current Simscape Interface/LConn2
  Series RLC Branch1/LConn1 -- Series RLC Branch4/RConn1 -- Voltage-Current Simscape Interface/LConn1
  V_battery+/RConn1 -- Series RLC Branch4/LConn1

== system battery_PV_microgrid/Microgrid Loads/Ideal Constant Resistance Load ==
  Bus Creator : BusCreator  Inputs=3  OutDataTypeStr=Bus: Load
  Current Measurement : powerlib/Measurements/Current Measurement  PhasorSimulation=off  OutputType=Complex  PSBequivalent=0
  Low-pass1 : TransferFcn  Numerator=100  Denominator=[1 100]
  Parallel RLC Branch : powerlib/Elements/Parallel RLC Branch  LConnTagsString=a  RConnTagsString=__new0  BranchType=R  Resistance=5  Inductance=1e-3  SetiL0=off  InitialCurrent=0  Capacitance=1e-6  Setx0=off  InitialVoltage=0  Measurements=None
  Product : Product
  V_load : powerlib/Measurements/Voltage Measurement  PhasorSimulation=off  OutputType=Complex  PSBequivalent=0
  V_P+ : PMIOPort  Port=1  Side=Left
  V_P- : PMIOPort  Port=2  Side=Left
  Load Measurements : Outport
  wires:
  Bus Creator/1 -> Load Measurements/1
  Product/1 -> Low-pass1/1
  V_load/1 -> Product/1, Bus Creator/1  "Voltage"
  Current Measurement/1 -> Product/2, Bus Creator/2  "Current"
  Low-pass1/1 -> Bus Creator/3  "Power"
  connections:
  V_load/LConn1 -- Current Measurement/LConn1 -- V_P+/RConn1
  Parallel RLC Branch/RConn1 -- V_load/LConn2 -- V_P-/RConn1
  Current Measurement/RConn1 -- Parallel RLC Branch/LConn1

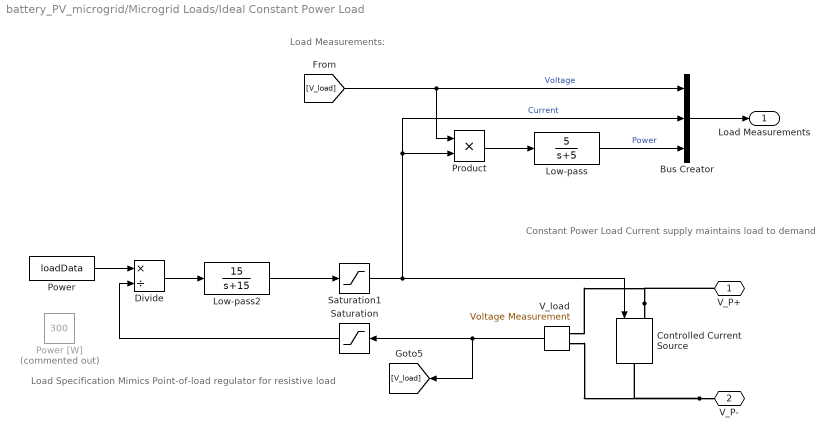
== system battery_PV_microgrid/Microgrid Loads/Ideal Constant Power Load ==
  note: Constant Power Load
      | Current supply maintains load to demand
  note: Load Measurements:
  note: Load Specification
      | Mimics Point-of-load regulator for resistive load
  Bus Creator : BusCreator  Inputs=3  OutDataTypeStr=Bus: Load
  Controlled Current Source : powerlib/Electrical Sources/Controlled Current Source  Initialize=on  Source_Type=AC  Amplitude=0  Phase=0  Frequency=0  Measurements=None
  Divide : Product  Inputs=*/
  Low-pass : TransferFcn  Numerator=[5]  Denominator=[1 5]
  Low-pass2 : TransferFcn  Numerator=[15]  Denominator=[1 15]
  Power : FromWorkspace  VariableName=loadData  SampleTime=0
  Power [W] : Constant  Commented=on  Value=300
  Product : Product
  Saturation : Saturate  UpperLimit=Inf  LowerLimit=5
  Saturation1 : Saturate  UpperLimit=30  LowerLimit=-Inf
  V_load : powerlib/Measurements/Voltage Measurement  PhasorSimulation=off  OutputType=Complex  PSBequivalent=0
  V_P+ : PMIOPort  Port=1  Side=Left
  V_P- : PMIOPort  Port=2  Side=Left
  Load Measurements : Outport
  wires:
  V_load/1 -> [V_load], Saturation/1
  Divide/1 -> Low-pass2/1
  Bus Creator/1 -> Load Measurements/1
  Product/1 -> Low-pass/1
  Low-pass/1 -> Bus Creator/3  "Power"
  Low-pass2/1 -> Saturation1/1
  Saturation/1 -> Divide/2
  Saturation1/1 -> Controlled Current Source/1, Bus Creator/2, Product/2  "Current"
  [V_load] -> Product/1, Bus Creator/1  "Voltage"
  Power/1 -> Divide/1
  connections:
  V_P-/RConn1 -- V_load/LConn2 -- Controlled Current Source/RConn1
  Controlled Current Source/LConn1 -- V_load/LConn1 -- V_P+/RConn1

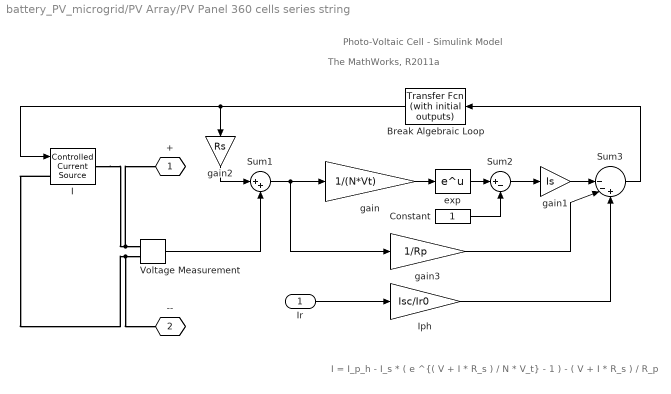
== system battery_PV_microgrid/PV Array/PV Panel 360 cells series string ==
  note: I = I_p_h - I_s * ( e ^{( V + I * R_s ) / N * V_t} - 1 ) - ( V + I * R_s ) / R_p
  note: Photo-Voltaic Cell - Simulink Model
  note: The MathWorks, R2011a
  Ir : Inport
  Break Algebraic Loop : simulink_extras/Additional Linear/Transfer Fcn (with initial outputs)  N=[1]  D="[tau  1]"  Y0=Isc  U0=0
  Constant : Constant
  I : powerlib/Electrical Sources/Controlled Current Source  Initialize=on  Source_Type=DC  Amplitude=5  Phase=0  Frequency=0  Measurements=None
  Iph : Gain  Gain=Isc/Ir0
  Sum1 : Sum  Inputs=|++
  Sum2 : Sum  Inputs=|+-
  Sum3 : Sum  Inputs=||--+
  Voltage Measurement : powerlib/Measurements/Voltage Measurement  PhasorSimulation=off  OutputType=Complex  PSBequivalent=0
  exp : Math  SaturateOnIntegerOverflow=on
  gain : Gain  Gain=1/(N*Vt)
  gain1 : Gain  Gain=Is
  gain2 : Gain  Gain=Rs
  gain3 : Gain  Gain=1/Rp
  + : PMIOPort  Tag=PMCPort  Port=1  Side=Right
  -- : PMIOPort  Tag=PMCPort  Port=2  Side=Right
  wires:
  Sum2/1 -> gain1/1
  Constant/1 -> Sum2/2
  exp/1 -> Sum2/1
  Sum1/1 -> gain/1, gain3/1
  gain/1 -> exp/1
  Sum3/1 -> Break Algebraic Loop/1
  Voltage Measurement/1 -> Sum1/2
  Ir/1 -> Iph/1
  Break Algebraic Loop/1 -> gain2/1, I/1
  gain2/1 -> Sum1/1
  gain1/1 -> Sum3/1
  gain3/1 -> Sum3/2
  Iph/1 -> Sum3/3
  connections:
  Voltage Measurement/LConn1 -- +/RConn1 -- I/RConn1
  Voltage Measurement/LConn2 -- --/RConn1 -- I/LConn1

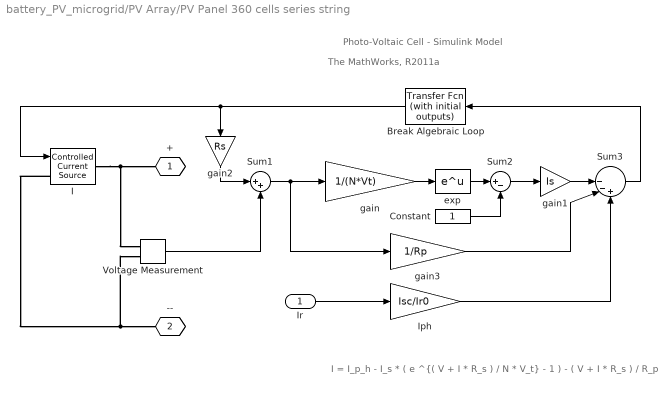
== system battery_PV_microgrid/PV Array/PV Panel 360 cells series string  ==
  note: The MathWorks, R2011a
  note: Photo-Voltaic Cell - Simulink Model
  note: I = I_p_h - I_s * ( e ^{( V + I * R_s ) / N * V_t} - 1 ) - ( V + I * R_s ) / R_p
  Ir : Inport
  Break Algebraic Loop : simulink_extras/Additional Linear/Transfer Fcn (with initial outputs)  N=[1]  D="[tau  1]"  Y0=Isc  U0=0
  Constant : Constant
  I : powerlib/Electrical Sources/Controlled Current Source  Initialize=on  Source_Type=DC  Amplitude=5  Phase=0  Frequency=0  Measurements=None
  Iph : Gain  Gain=Isc/Ir0
  Sum1 : Sum  Inputs=|++
  Sum2 : Sum  Inputs=|+-
  Sum3 : Sum  Inputs=||--+
  Voltage Measurement : powerlib/Measurements/Voltage Measurement  PhasorSimulation=off  OutputType=Complex  PSBequivalent=0
  exp : Math  SaturateOnIntegerOverflow=on
  gain : Gain  Gain=1/(N*Vt)
  gain1 : Gain  Gain=Is
  gain2 : Gain  Gain=Rs
  gain3 : Gain  Gain=1/Rp
  + : PMIOPort  Tag=PMCPort  Port=1  Side=Right
  -- : PMIOPort  Tag=PMCPort  Port=2  Side=Right
  wires:
  Iph/1 -> Sum3/3
  gain3/1 -> Sum3/2
  gain1/1 -> Sum3/1
  gain2/1 -> Sum1/1
  Break Algebraic Loop/1 -> I/1, gain2/1
  Ir/1 -> Iph/1
  Voltage Measurement/1 -> Sum1/2
  Sum3/1 -> Break Algebraic Loop/1
  gain/1 -> exp/1
  Sum1/1 -> gain3/1, gain/1
  exp/1 -> Sum2/1
  Constant/1 -> Sum2/2
  Sum2/1 -> gain1/1
  connections:
  I/LConn1 -- --/RConn1 -- Voltage Measurement/LConn2
  I/RConn1 -- +/RConn1 -- Voltage Measurement/LConn1

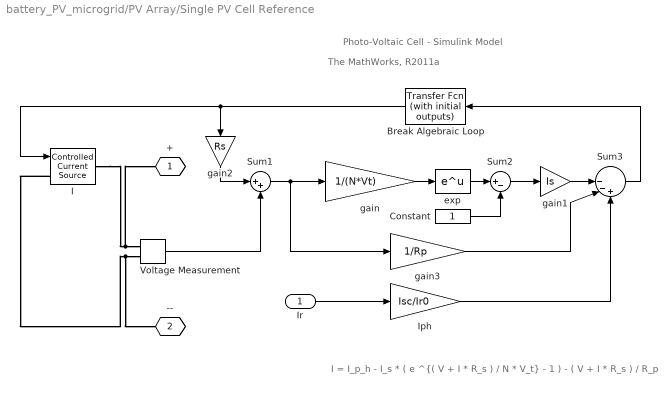
== system battery_PV_microgrid/PV Array/Single PV Cell Reference ==
  note: I = I_p_h - I_s * ( e ^{( V + I * R_s ) / N * V_t} - 1 ) - ( V + I * R_s ) / R_p
  note: Photo-Voltaic Cell - Simulink Model
  note: The MathWorks, R2011a
  Ir : Inport
  Break Algebraic Loop : simulink_extras/Additional Linear/Transfer Fcn (with initial outputs)  N=[1]  D="[tau  1]"  Y0=Isc  U0=0
  Constant : Constant
  I : powerlib/Electrical Sources/Controlled Current Source  Initialize=on  Source_Type=DC  Amplitude=5  Phase=0  Frequency=0  Measurements=None
  Iph : Gain  Gain=Isc/Ir0
  Sum1 : Sum  Inputs=|++
  Sum2 : Sum  Inputs=|+-
  Sum3 : Sum  Inputs=||--+
  Voltage Measurement : powerlib/Measurements/Voltage Measurement  PhasorSimulation=off  OutputType=Complex  PSBequivalent=0
  exp : Math  SaturateOnIntegerOverflow=on
  gain : Gain  Gain=1/(N*Vt)
  gain1 : Gain  Gain=Is
  gain2 : Gain  Gain=Rs
  gain3 : Gain  Gain=1/Rp
  + : PMIOPort  Tag=PMCPort  Port=1  Side=Right
  -- : PMIOPort  Tag=PMCPort  Port=2  Side=Right
  wires:
  Sum2/1 -> gain1/1
  Constant/1 -> Sum2/2
  exp/1 -> Sum2/1
  Sum1/1 -> gain/1, gain3/1
  gain/1 -> exp/1
  Sum3/1 -> Break Algebraic Loop/1
  Voltage Measurement/1 -> Sum1/2
  Ir/1 -> Iph/1
  Break Algebraic Loop/1 -> gain2/1, I/1
  gain2/1 -> Sum1/1
  gain1/1 -> Sum3/1
  gain3/1 -> Sum3/2
  Iph/1 -> Sum3/3
  connections:
  Voltage Measurement/LConn1 -- +/RConn1 -- I/RConn1
  Voltage Measurement/LConn2 -- --/RConn1 -- I/LConn1

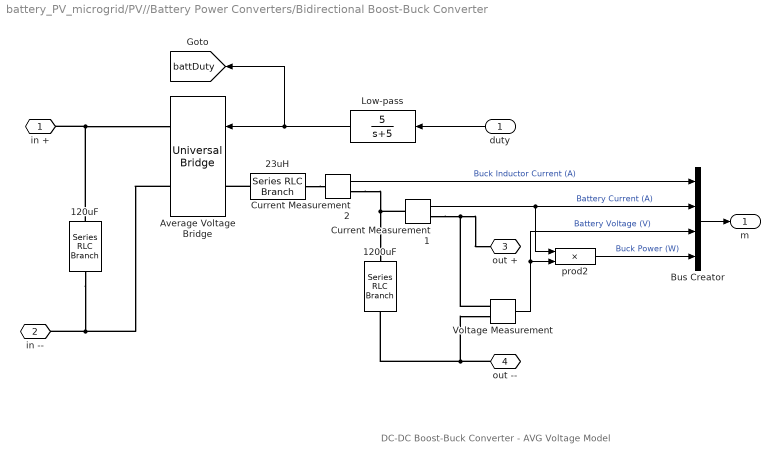
== system battery_PV_microgrid/PV//Battery Power Converters/Bidirectional Boost-Buck Converter ==
  note: DC-DC Boost-Buck Converter - AVG Voltage Model
  duty : Inport
  1200uF : powerlib/Elements/Series RLC Branch  LConnTagsString=__new0  RConnTagsString=__new0  BranchType=RC  Resistance=0.05  Inductance=30e-6  SetiL0=off  InitialCurrent=0  Capacitance=120e-6  Setx0=on  InitialVoltage=24  Measurements=None
  "120uF " : powerlib/Elements/Series RLC Branch  LConnTagsString=__new0  RConnTagsString=__new0  BranchType=RC  Resistance=0.005  Inductance=30e-6  SetiL0=off  InitialCurrent=0  Capacitance=120e-6  Setx0=on  InitialVoltage=30  Measurements=None
  23uH : powerlib/Elements/Series RLC Branch  LConnTagsString=__new0  RConnTagsString=__new0  BranchType=RL  Resistance=0.01  Inductance=23e-6  SetiL0=off  InitialCurrent=16.1  Capacitance=1e-6  Setx0=off  InitialVoltage=0  Measurements=None
  Average Voltage Bridge : powerlib/Power Electronics/Universal Bridge  Arms=1  SnubberResistance=1e5  SnubberCapacitance=inf  Device=Average-model based VSC  Ron=1e-4  Lon=0  ForwardVoltages="[  0  0  ]"  ForwardVoltage=0  GTOparameters=[ 10e-6 , 20e-6 ]  IGBTparameters=[ 1e-6 , 2e-6 ]  Measurements=None  Measurements_2=None  converterType=Rectifier
  Bus Creator : BusCreator
  Current Measurement1 : powerlib/Measurements/Current Measurement  PhasorSimulation=off  OutputType=Complex  PSBequivalent=0
  Current Measurement2 : powerlib/Measurements/Current Measurement  PhasorSimulation=off  OutputType=Complex  PSBequivalent=0
  Low-pass : TransferFcn  Numerator=5  Denominator=[1 5]
  Voltage Measurement : powerlib/Measurements/Voltage Measurement  PhasorSimulation=off  OutputType=Complex  PSBequivalent=0
  prod2 : Product  Inputs=**
  in + : PMIOPort  Port=1  Side=Left
  in -- : PMIOPort  Port=2  Side=Left
  out + : PMIOPort  Port=3  Side=Right
  out -- : PMIOPort  Port=4  Side=Right
  m : Outport
  tag scope: battDuty=global
  wires:
  prod2/1 -> Bus Creator/4  "Buck Power (W)"
  Current Measurement2/1 -> Bus Creator/1  "Buck Inductor Current (A)"
  Current Measurement1/1 -> prod2/1, Bus Creator/2  "Battery Current (A)"
  Voltage Measurement/1 -> prod2/2, Bus Creator/3  "Battery Voltage (V)"
  Bus Creator/1 -> m/1
  duty/1 -> Low-pass/1
  Low-pass/1 -> [battDuty], Average Voltage Bridge/1
  connections:
  Voltage Measurement/LConn1 -- out +/RConn1 -- Current Measurement1/RConn1
  "120uF "/LConn1 -- Average Voltage Bridge/RConn1 -- in +/RConn1
  Average Voltage Bridge/RConn2 -- in --/RConn1 -- "120uF "/RConn1
  23uH/RConn1 -- Average Voltage Bridge/LConn1
  out --/RConn1 -- 1200uF/RConn1 -- Voltage Measurement/LConn2
  Current Measurement1/LConn1 -- 1200uF/LConn1 -- Current Measurement2/RConn1
  23uH/LConn1 -- Current Measurement2/LConn1

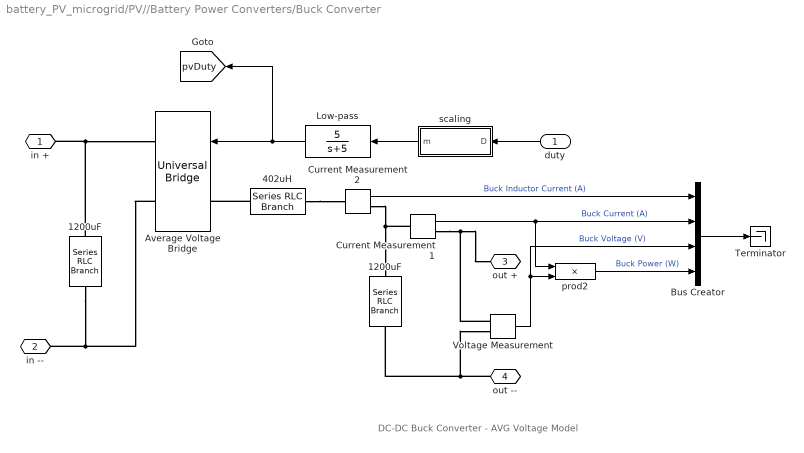
== system battery_PV_microgrid/PV//Battery Power Converters/Buck Converter ==
  note: DC-DC Buck Converter - AVG Voltage Model
  duty : Inport
  1200uF : powerlib/Elements/Series RLC Branch  LConnTagsString=__new0  RConnTagsString=__new0  BranchType=RC  Resistance=0.25  Inductance=30e-6  SetiL0=off  InitialCurrent=0  Capacitance=1200e-6  Setx0=on  InitialVoltage=30  Measurements=None
  "1200uF " : powerlib/Elements/Series RLC Branch  LConnTagsString=__new0  RConnTagsString=__new0  BranchType=RC  Resistance=0.25  Inductance=30e-6  SetiL0=off  InitialCurrent=0  Capacitance=1200e-6  Setx0=on  InitialVoltage=53  Measurements=None
  402uH : powerlib/Elements/Series RLC Branch  LConnTagsString=__new0  RConnTagsString=__new0  BranchType=RL  Resistance=0.001  Inductance=402e-6  SetiL0=off  InitialCurrent=-14  Capacitance=1e-6  Setx0=off  InitialVoltage=0  Measurements=None
  Average Voltage Bridge : powerlib/Power Electronics/Universal Bridge  Arms=1  SnubberResistance=1e5  SnubberCapacitance=inf  Device=Average-model based VSC  Ron=1e-4  Lon=0  ForwardVoltages="[  0  0  ]"  ForwardVoltage=0  GTOparameters=[ 10e-6 , 20e-6 ]  IGBTparameters=[ 1e-6 , 2e-6 ]  Measurements=None  Measurements_2=None  converterType=Rectifier
  Bus Creator : BusCreator
  Current Measurement1 : powerlib/Measurements/Current Measurement  PhasorSimulation=off  OutputType=Complex  PSBequivalent=0
  Current Measurement2 : powerlib/Measurements/Current Measurement  PhasorSimulation=off  OutputType=Complex  PSBequivalent=0
  Low-pass : TransferFcn  Numerator=5  Denominator=[1 5]
  Terminator : Terminator
  Voltage Measurement : powerlib/Measurements/Voltage Measurement  PhasorSimulation=off  OutputType=Complex  PSBequivalent=0
  prod2 : Product  Inputs=**
  scaling : Subsystem
  in + : PMIOPort  Port=1  Side=Left
  in -- : PMIOPort  Port=2  Side=Left
  out + : PMIOPort  Port=3  Side=Right
  out -- : PMIOPort  Port=4  Side=Right
  tag scope: pvDuty=global
  wires:
  prod2/1 -> Bus Creator/4  "Buck Power (W)"
  duty/1 -> scaling/1(D)
  Current Measurement2/1 -> Bus Creator/1  "Buck Inductor Current (A)"
  Current Measurement1/1 -> prod2/1, Bus Creator/2  "Buck Current (A)"
  Voltage Measurement/1 -> prod2/2, Bus Creator/3  "Buck Voltage (V)"
  Bus Creator/1 -> Terminator/1
  scaling/1(m) -> Low-pass/1
  Low-pass/1 -> [pvDuty], Average Voltage Bridge/1
  connections:
  Voltage Measurement/LConn1 -- out +/RConn1 -- Current Measurement1/RConn1
  "1200uF "/LConn1 -- Average Voltage Bridge/RConn1 -- in +/RConn1
  Average Voltage Bridge/RConn2 -- in --/RConn1 -- "1200uF "/RConn1
  402uH/RConn1 -- Average Voltage Bridge/LConn1
  out --/RConn1 -- 1200uF/RConn1 -- Voltage Measurement/LConn2
  Current Measurement1/LConn1 -- Current Measurement2/RConn1 -- 1200uF/LConn1
  402uH/LConn1 -- Current Measurement2/LConn1

== system battery_PV_microgrid/PV//Battery Power Converters/Calculate Power ==
  meas_converter : Inport
  Bus Selector : BusSelector  OutputSignals=Battery Voltage (V),Battery Current (A)
  Low-pass : TransferFcn  Numerator=[5]  Denominator=[1 5]
  Product : Product
  power : Outport
  voltage : Outport  Port=2
  current : Outport  Port=3
  wires:
  meas_converter/1 -> Bus Selector/1
  Bus Selector/1 -> voltage/1, Product/1  "<Battery Voltage (V)>"
  Bus Selector/2 -> current/1, Product/2  "<Battery Current (A)>"
  Product/1 -> Low-pass/1
  Low-pass/1 -> power/1

== system battery_PV_microgrid/Scopes/Unpack Battery Signals ==
  Measure : Inport
  Bus Selector : BusSelector  OutputSignals=batt.Voltage,batt.Current,batt.SOC,batt.Temperature
  Voltage : Outport
  Current : Outport  Port=2
  SOC : Outport  Port=3
  Temperature : Outport  Port=4
  wires:
  Bus Selector/2 -> Current/1  "<Current>"
  Measure/1 -> Bus Selector/1
  Bus Selector/1 -> Voltage/1  "<Voltage>"
  Bus Selector/3 -> SOC/1  "<SOC>"
  Bus Selector/4 -> Temperature/1  "<Temperature>"

== system battery_PV_microgrid/Scopes/Unpack PV Signals ==
  Measure : Inport
  Bus Selector : BusSelector  OutputSignals=pv.Voltage,pv.Current
  Voltage : Outport
  Current : Outport  Port=2
  wires:
  Bus Selector/1 -> Voltage/1  "<Voltage>"
  Measure/1 -> Bus Selector/1
  Bus Selector/2 -> Current/1  "<Current>"

== system battery_PV_microgrid/Scopes/Unpack Power Signals ==
  Measure : Inport
  Bus Selector : BusSelector  OutputSignals=load.Power,pv.Power,bus.BattPower,grid.power
  Negate : Gain  Gain=-1
  Load : Outport
  PV : Outport  Port=2
  Battery : Outport  Port=3
  Grid : Outport  Port=4
  wires:
  Measure/1 -> Bus Selector/1
  Bus Selector/3 -> Negate/1  "<BattPower>"
  Bus Selector/4 -> Grid/1  "<power>"
  Negate/1 -> Battery/1
  Bus Selector/1 -> Load/1  "<Power>"
  Bus Selector/2 -> PV/1  "<Power>"
